simulink model "weightloss"  (R2022a)
settings: Solver=VariableStepAuto  StartTime=0.0  StopTime=3000  RelTol=1e-3
libraries: cstblocks x1
settings Model: Creator=anthony  LastModifiedBy=anthony

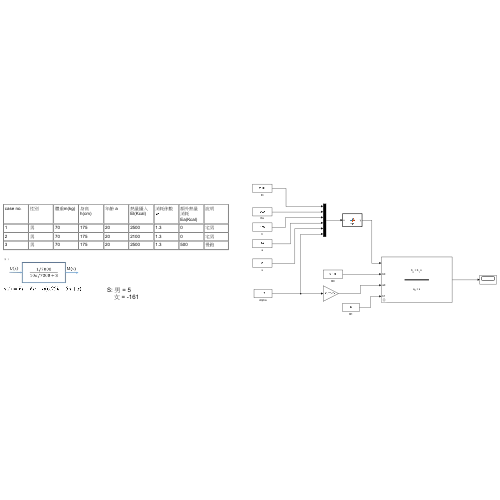
[thumbnail: Simulink's stored preview of the top-level diagram]
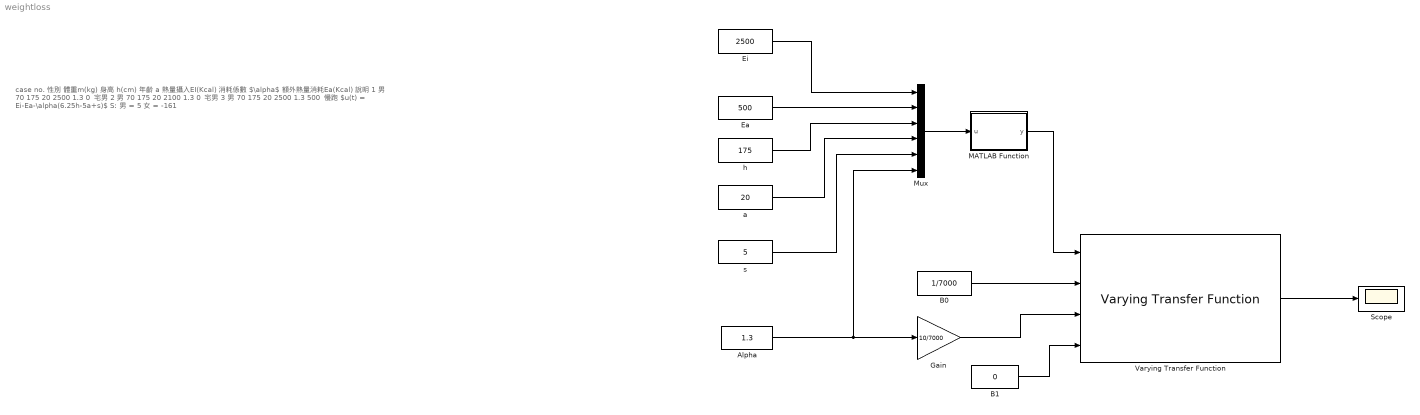
== system weightloss ==
  note: case no.
      | 性別
      | 體重m(kg)
      | 身高
      | h(cm)
      | 年齡 a
      | 熱量攝入EI(Kcal)
      | 消耗係數
      | $\alpha$
      | 額外熱量消耗Ea(Kcal)
      | 說明
      |
      | 1
      | 男
      | 70
      | 175
      | 20
      | 2500
      | 1.3
      | 0
      | 宅男
      |
      | 2
      | 男
      | 70
      | 175
      | 20
      | 2100
      | 1.3
      | 0
      | 宅男
      |
      | 3
      | 男
      | 70
      | 175
      | 20
      | 2500
      | 1.3
      | 500
      | 慢跑
      |
      | $u(t) = Ei-Ea-\alpha(6.25h-5a+s)$ S: 男 = 5
      | 女 = -161
  Alpha : Constant  Value=1.3
  B0 : Constant  Value=1/7000
  B1 : Constant  Value=0
  Ea : Constant  Value=500
  Ei : Constant  Value=2500
  Gain : Gain  Gain=10/7000
  MATLAB Function : MATLAB Function  TreatAsAtomicUnit=on
  Mux : Mux  Inputs=6
  Scope : Scope
  Varying Transfer Function : cstblocks/Linear Parameter Varying/Varying Transfer Function  N=1
      link override Integrator1: InitialCondition=70
  a : Constant  Value=20
  h : Constant  Value=175
  s : Constant  Value=5
  wires:
  B1/1 -> Varying Transfer Function/4
  B0/1 -> Varying Transfer Function/2
  Alpha/1 -> Mux/6, Gain/1
  Gain/1 -> Varying Transfer Function/3
  Ei/1 -> Mux/1
  Ea/1 -> Mux/2
  h/1 -> Mux/3
  a/1 -> Mux/4
  s/1 -> Mux/5
  Mux/1 -> MATLAB Function/1(u)
  Varying Transfer Function/1 -> Scope/1
  MATLAB Function/1(y) -> Varying Transfer Function/1

== matlab function weightloss/MATLAB Function ==
  data: u input; y output
function y = fcn(u)
y = u(1) - u(2) - u(6)*(6.25*u(3)-5*u(4)+u(5));
